simulink subsystem "SelfDefined_Half_Bridge_Converter"  (R2024b)
settings: Solver=VariableStepAuto  StartTime=0.0  StopTime=10.0  RelTol=1e-3
libraries: spsIGBTDiodeLib x2, simulink x1
settings Model: Creator=XixiLab  LastModifiedBy=XixiLab

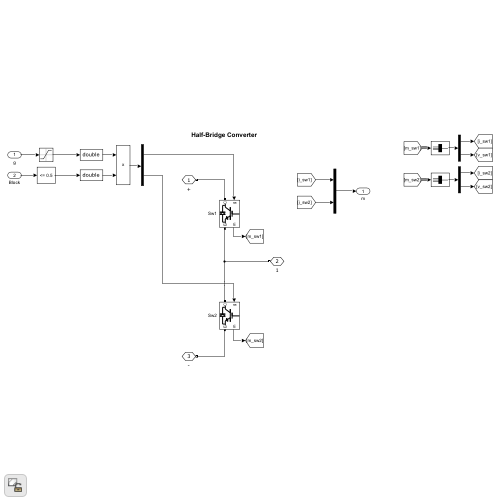
[thumbnail: Simulink's stored preview of the top-level diagram]
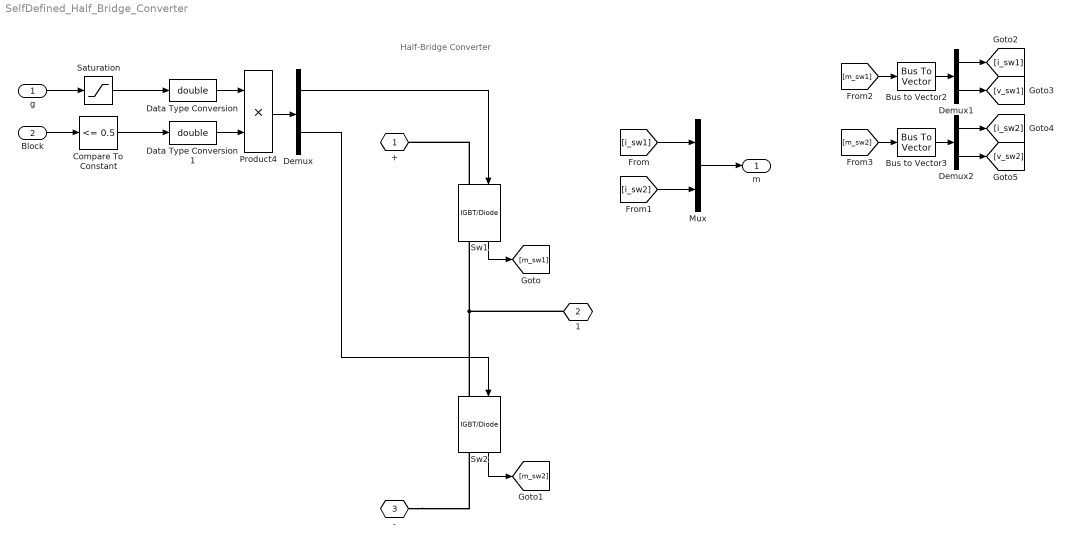
== system SelfDefined_Half_Bridge_Converter ==
  note: Half-Bridge Converter
  g : Inport  PortDimensions=2
  Block : Inport  Port=2  PortDimensions=1
  Bus to Vector2 : BusToVector
  Bus to Vector3 : BusToVector
  Compare To Constant : simulink/Logic and Bit Operations/Compare To Constant  relop=<=  const=0.5  OutDataTypeStr=boolean
  Data Type Conversion : DataTypeConversion  OutDataTypeStr=double  SaturateOnIntegerOverflow=off  RndMeth=Floor
  Data Type Conversion1 : DataTypeConversion  OutDataTypeStr=double  SaturateOnIntegerOverflow=off  RndMeth=Floor
  Demux : Demux  Outputs=2
  Demux1 : Demux  Outputs=2
  Demux2 : Demux  Outputs=2
  Mux : Mux  Inputs=2
  Product4 : Product
  Saturation : Saturate  UpperLimit=1  LowerLimit=0
  Sw1 : spsIGBTDiodeLib/IGBT//Diode  Ron=1e-3  Rs=1e6  Cs=inf  Measurements=on
  Sw2 : spsIGBTDiodeLib/IGBT//Diode  Ron=1e-3  Rs=1e6  Cs=inf  Measurements=on
  + : PMIOPort  Tag=PMCPort  Side=Right
  1 : PMIOPort  Tag=PMCPort  Port=2  Side=Left
  - : PMIOPort  Tag=PMCPort  Port=3  Side=Right
  m : Outport
  wires:
  Product4/1 -> Demux/1
  Data Type Conversion/1 -> Product4/1
  Demux/2 -> Sw2/1
  Data Type Conversion1/1 -> Product4/2
  Block/1 -> Compare To Constant/1
  Saturation/1 -> Data Type Conversion/1
  g/1 -> Saturation/1
  Compare To Constant/1 -> Data Type Conversion1/1
  Demux/1 -> Sw1/1
  Sw1/1 -> [m_sw1]
  Sw2/1 -> [m_sw2]
  Mux/1 -> m/1
  [i_sw1] -> Mux/1
  [i_sw2] -> Mux/2
  [m_sw1] -> Bus to Vector2/1
  Bus to Vector2/1 -> Demux1/1
  Demux1/1 -> [i_sw1]
  Demux1/2 -> [v_sw1]
  Demux2/2 -> [v_sw2]
  Demux2/1 -> [i_sw2]
  [m_sw2] -> Bus to Vector3/1
  Bus to Vector3/1 -> Demux2/1
  connections:
  1/RConn1 -- Sw2/LConn1 -- Sw1/RConn1
  -/RConn1 -- Sw2/RConn1
  Sw1/LConn1 -- +/RConn1
